simulink model "test_asynchronous_machines"  (R2025b)
settings: Solver=VariableStepAuto  StartTime=0.0  StopTime=20  RelTol=1e-3
libraries: ee_lib x3, ee_lib_for_power_systems x3, fl_lib x1, nesl_utility x1
settings Model: SimulationMode=accelerator  Creator=gdudgeon  LastModifiedBy=gdudgeon
settings RTWCC: GPUComputeCapability=3.5

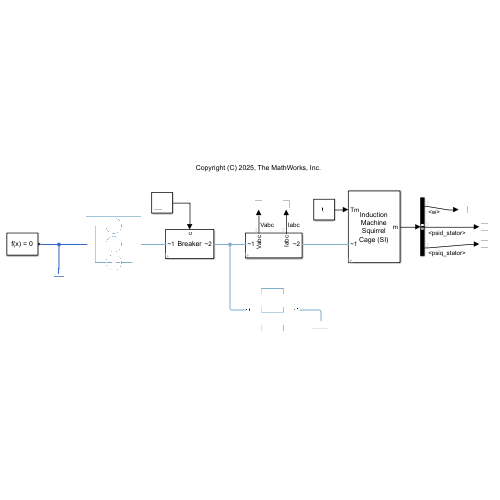
[thumbnail: Simulink's stored preview of the top-level diagram]
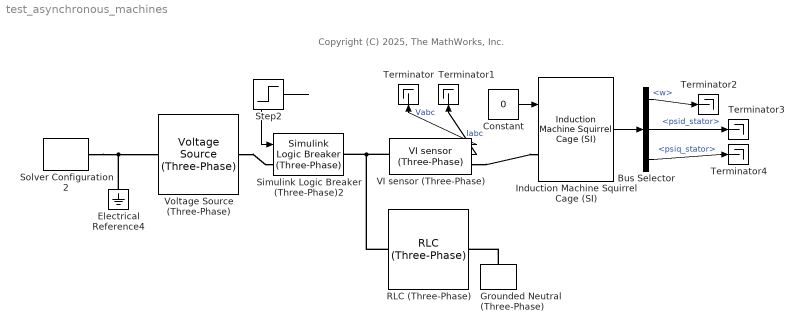
== system test_asynchronous_machines ==
  note: Copyright (C) 2025, The MathWorks, Inc.
  Bus Selector : BusSelector  OutputSignals=w,psid_stator,psiq_stator
  Constant : Constant  Value=0
  Electrical Reference4 : fl_lib/Electrical/Electrical Elements/Electrical Reference
  Grounded Neutral (Three-Phase) : ee_lib/Connectors & References/Grounded Neutral (Three-Phase)
  Induction Machine Squirrel Cage (SI) : ee_lib_for_power_systems/Electromechanical Machines/Induction Machine Squirrel Cage (SI)  run_time=off  Pnom=15e3  Vnom=220  Fnom=60  p=1  Rs=0.25  Xls=0.4  Rrp=0.14  Xlrp=0.41  Xm=17  J=1
      link override Subsystem/Gain: Gain=2*pi*Fnom
      settings: SourceProductName=Support Library for Power Systems
  RLC (Three-Phase) : ee_lib/Passive/RLC Assemblies/RLC (Three-Phase)  port_option=ee.enum.threePhasePort.composite  component_structure=ee.enum.rlc.structure.R  R=10 Ohm  L=1e-3 H  C=1e-6 F  R_parasitic=0 Ohm  G_parasitic=0 1/Ohm  IL_specify=off  IL_priority=High  IL=[0, 0, 0] A  IL_nominal_specify=off  IL_nominal_value=1  IL_nominal_unit=A  VC_specify=off  VC_priority=High  VC=[0, 0, 0] V  VC_nominal_specify=off  VC_nominal_value=1  VC_nominal_unit=V
      settings: InternalSimscapePortConfiguration="{\"Bottom\":[],\"Left\":[{\"id\":\"N1\",\"label\":\"~1\",\"type\":\"foundation.electrical.three_phase\"}],\"Right\":[{\"id\":\"N2\",\"label\":\"~2\",\"type\":\"foundation.electrical.three_phase\"}],\"Top\":[]}"
  Simulink Logic Breaker (Three-Phase)2 : ee_lib_for_power_systems/Network Components/Simulink Logic Breaker (Three-Phase)  initB=0  Ron=1e-3  Goff=1e-3  Ts=5e-5
      settings: SourceProductName=Support Library for Power Systems
  Solver Configuration 2 : nesl_utility/Solver Configuration  PhysicalDomain=network_engine_domain  SubClassName=solver  LeftPortType=input  RightPortType=generic  Tones=[]  Harmonics=[]  SimulateNoise=off  Profile=off  UseLocalSampling=off  EnableSwitchedLinearOptims=on  FrequencyDomain=off  UseCCode=off  RelTol=0.001  AbsTol=0.001  MinStep=1e-09  ToWorkspace=off  RevertToSquareIcSolve=off  NumHomotopyIterations=100  PhasorMode=off  PhasorModeNumHarmonics=1  ConsistencySolver=NEWTON_XTOL_AFTER_FTOL  IndexReductionMethod=None  DoDC=off  ResidualTolerance=1e-09  ConsistencyTolSource=GLOBAL  ConsistencyAbsTol=0.001  ConsistencyRelTol=0.001  ConsistencyTolFactor=0.001  UseLocalSolver=on  LocalSolverChoice=NE_PARTITIONING_ADVANCER  ResolveIndetEquations=off  FunctionEvalNumThread=1  LocalSolverSampleTime=50e-6  DoFixedCost=off  MaxNonlinIter=2  MaxModeIter=2  ComputeImpulses=off  ImpulseIterations=2  LinearAlgebra=Sparse  LinearAlgebraNumThread=0  EquationFormulation=NE_TIME_EF  DelaysMemoryBudget=1024  AutomaticFiltering=off  FilteringTimeConstant=0.001  PartitionStorageMethod=AS_NEEDED  PartitionMemoryBudget=1024  PartitionMethod=ROBUST  MultibodyUseLocalSolver=off  MultibodyLocalSolverChoice=ODE1  MultibodyLocalSolverSampleTime=0.001
  Step2 : Step  Time=2  SampleTime=5e-5
  Terminator{,1..4} (5 alike) : Terminator
  VI sensor (Three-Phase) : ee_lib_for_power_systems/Sense and Measure/VI sensor (Three-Phase)  volt_meas=Phase-to-Ground (Phase Voltage)  meas_units=SI  Vnom=24e3  Pnom=100e6
      settings: SourceProductName=Support Library for Power Systems
  Voltage Source (Three-Phase) : ee_lib/Sources/Voltage Source (Three-Phase)  vline_rms=220 V  shift=0 deg  freq=60 Hz  impedance_option=0  SShortCircuit=1e6 A*V  XR=15  R=0.01 Ohm  L=3.97e-4 H  harmonic_option=0  harmonic_orders=[5, 7, 11, 13]  harmonic_ratios=[.1, .1, .1, .1]  G_parasitic=0 1/Ohm  I_specify=off  I_priority=None  I=[0, 0, 0] A  I_nominal_specify=off  I_nominal_value=1  I_nominal_unit=A
  wires:
  Step2/1 -> Simulink Logic Breaker (Three-Phase)2/1
  VI sensor (Three-Phase)/1 -> Terminator/1  "Vabc"
  VI sensor (Three-Phase)/2 -> Terminator1/1  "Iabc"
  Induction Machine Squirrel Cage (SI)/1 -> Bus Selector/1
  Bus Selector/1 -> Terminator2/1  "<w>"
  Constant/1 -> Induction Machine Squirrel Cage (SI)/1
  Bus Selector/2 -> Terminator3/1  "<psid_stator>"
  Bus Selector/3 -> Terminator4/1  "<psiq_stator>"
  connections:
  Voltage Source (Three-Phase)/RConn1 -- Simulink Logic Breaker (Three-Phase)2/LConn1
  Electrical Reference4/LConn1 -- Voltage Source (Three-Phase)/LConn1 -- Solver Configuration 2/RConn1
  VI sensor (Three-Phase)/LConn1 -- RLC (Three-Phase)/LConn1 -- Simulink Logic Breaker (Three-Phase)2/RConn1
  VI sensor (Three-Phase)/RConn1 -- Induction Machine Squirrel Cage (SI)/LConn1
  Grounded Neutral (Three-Phase)/LConn1 -- RLC (Three-Phase)/RConn1
